simulink model "IfElseIfElse"  (R2020a)
settings: Solver=FixedStepDiscrete  StartTime=0.0  StopTime=30  FixedStep=0.1  RelTol=1e-3
settings Model: Creator=ashok  LastModifiedBy=ashok
settings DataIOCC: ExternalInput=[t, y]  LoadExternalInput=on

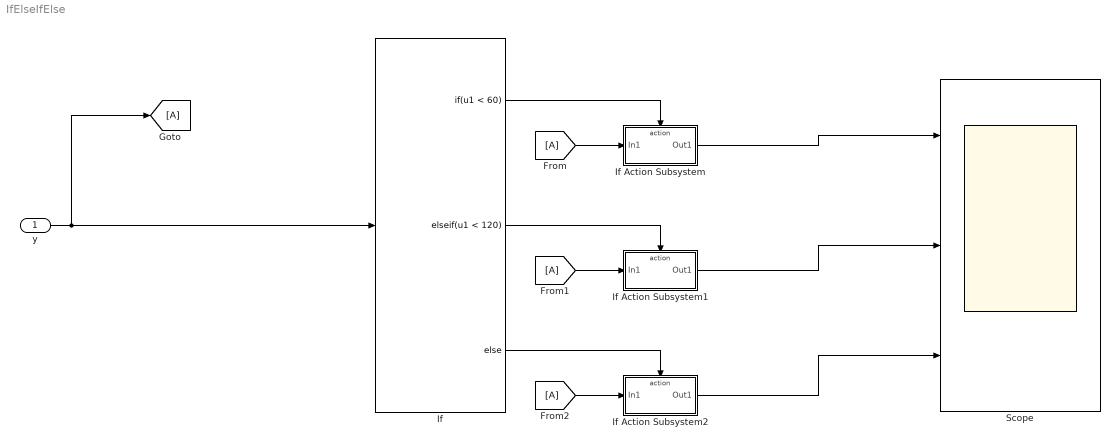
== system IfElseIfElse ==
  y : Inport
  If : If  IfExpression=u1 < 60  ElseIfExpressions=u1 < 120
  If Action Subsystem : Subsystem  TreatAsAtomicUnit=on
  If Action Subsystem1 : Subsystem  TreatAsAtomicUnit=on
  If Action Subsystem2 : Subsystem  TreatAsAtomicUnit=on
  Scope : Scope  NumInputPorts=3
  wires:
  y/1 -> If/1, [A]
  If/1 -> If Action Subsystem/Action
  [A] -> If Action Subsystem/1(In1)
  If/2 -> If Action Subsystem1/Action
  [A] -> If Action Subsystem1/1(In1)
  [A] -> If Action Subsystem2/1(In1)
  If/3 -> If Action Subsystem2/Action
  If Action Subsystem/1(Out1) -> Scope/1
  If Action Subsystem1/1(Out1) -> Scope/2
  If Action Subsystem2/1(Out1) -> Scope/3

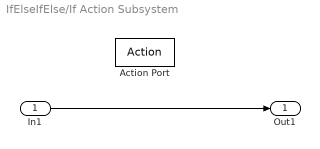
== system IfElseIfElse/If Action Subsystem ==
  In1 : Inport
  Action Port : ActionPort  ActionPortLabel=if(u1 < 60)
  Out1 : Outport
  wires:
  In1/1 -> Out1/1

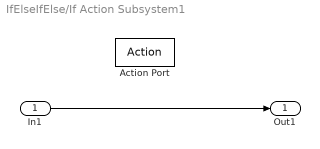
== system IfElseIfElse/If Action Subsystem1 ==
  In1 : Inport
  Action Port : ActionPort  ActionPortLabel=elseif(u1 < 120)
  Out1 : Outport
  wires:
  In1/1 -> Out1/1

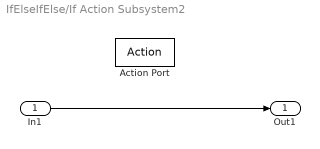
== system IfElseIfElse/If Action Subsystem2 ==
  In1 : Inport
  Action Port : ActionPort  ActionPortLabel=else
  Out1 : Outport
  wires:
  In1/1 -> Out1/1
